simulink model "lab2_2"  (Simulink 7.9)
settings: Solver=ode45  StartTime=0.0  StopTime=1  RelTol=1e-3
libraries: simulink x1
settings Model: Creator=Aquirel  LastModifiedBy=Aquirel

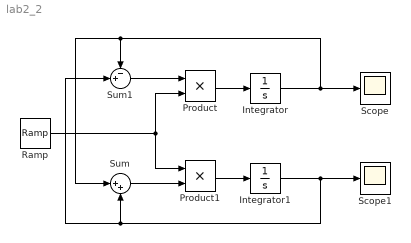
== system lab2_2 ==
  Integrator : Integrator  InitialCondition=1
  Integrator1 : Integrator  InitialCondition=1
  Product : Product  RndMeth=Zero
  Product1 : Product  RndMeth=Zero
  Ramp : simulink/Sources/Ramp  slope=1  start=0  X0=0
  Scope : Scope
      settings: YMin=0  YMax=2.5
  Scope1 : Scope
      settings: YMin=0  YMax=2.5
  Sum : Sum  Inputs=|++
  Sum1 : Sum  Inputs=-+|
  wires:
  Sum1/1 -> Product/1
  Ramp/1 -> Product1/1, Product/2
  Product/1 -> Integrator/1
  Integrator/1 -> Scope/1, Sum/1, Sum1/1
  Sum/1 -> Product1/2
  Product1/1 -> Integrator1/1
  Integrator1/1 -> Scope1/1, Sum/2, Sum1/2
